simulink model "RealtimeModel"  (Simulink 7.0)
settings: Solver=FixedStepDiscrete  SolverMode=MultiTasking  StartTime=0.0  StopTime=RunningTime  FixedStep=sample  RelTol=1e-3
undefined symbols (not defined in the file): Elements, Integrator, SampleRate, Structure
libraries: simulink x2
(part 1 of 3)
settings Model: Creator=Tommy  LastModifiedBy=Tommy  BufferReuse=off
settings OptimizationCC: BlockReduction=off  OptimizeBlockIOStorage=off  BufferReuse=off  ExpressionFolding=off  LocalBlockOutputs=off
settings RTWCC: SystemTargetFile=xpctarget.tlc  TemplateMakefile=xpc_default_tmf  Description=xPC Target  ProcessScript=xpctarget_make_rtw_hook
settings xpcTargetCC: TargetFcnLib=ansi_tfl_table_tmw.mat  GenFloatMathFcnCalls=ANSI_C  CompOptLevelCompliant=off  PortableWordSizes=off
settings CustomProperty: DataType=string  Value=Real-Time

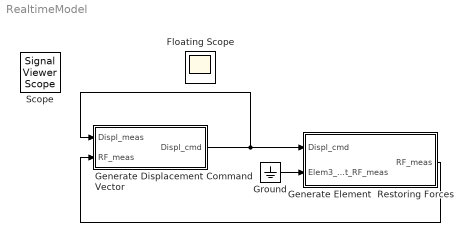
== system RealtimeModel ==
  Generate Displacement Command Vector : Subsystem
      mask Type: Generate Displacement Command Vector
      mask Description:
      | Generates the Displacement vector using the CR Algorithm.
      | 
      | Connect the measured displacement vector and measured restoring force vector to the inputs.
  Generate Element  Restoring Forces : Subsystem  TreatAsAtomicUnit=on  SystemSampleTime=SampleRate
  Ground : Ground
  Floating Scope : Scope
      settings: Floating=on
  Scope : SignalViewerScope  IOType=viewer  SampleTime=-1  RefreshTime=0.035000
  wires:
  Generate Displacement Command Vector/1(Displ_cmd) -> Generate Element  Restoring Forces/1(Displ_cmd), Generate Displacement Command Vector/1(Displ_meas)
  Generate Element  Restoring Forces/1(RF_meas) -> Generate Displacement Command Vector/2(RF_meas)
  Ground/1 -> Generate Element  Restoring Forces/2(Elem3_Act_RF_meas)

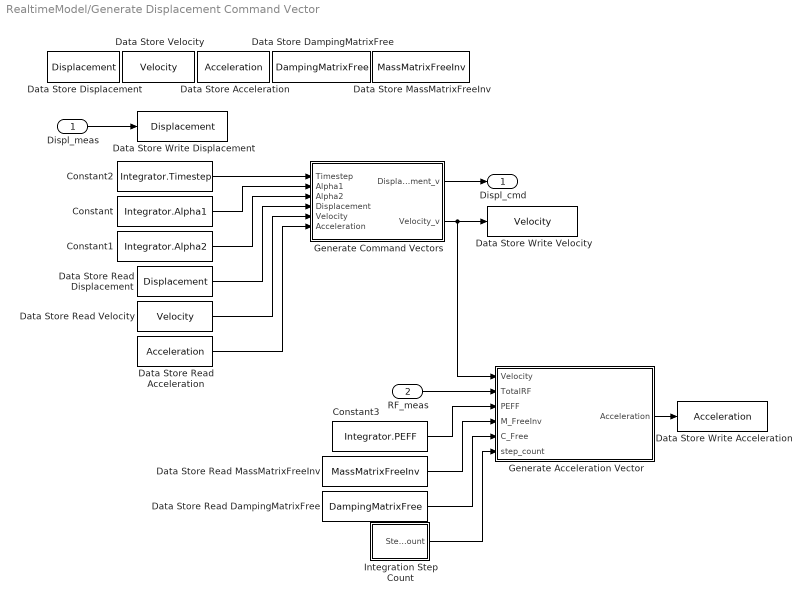
== system RealtimeModel/Generate Displacement Command Vector ==
  Displ_meas : Inport  OutDataType=sfix(16)  OutScaling=2^0
  RF_meas : Inport  Port=2  OutDataType=sfix(16)  OutScaling=2^0
  Constant : Constant  Value=Integrator.Alpha1  OutDataType=sfix(16)  OutScaling=2^0
  Constant1 : Constant  Value=Integrator.Alpha2  OutDataType=sfix(16)  OutScaling=2^0
  Constant2 : Constant  Value=Integrator.Timestep  OutDataType=sfix(16)  OutScaling=2^0
  Constant3 : Constant  Value=Integrator.PEFF  OutDataType=sfix(16)  OutScaling=2^0
  Data Store Acceleration : DataStoreMemory  DataStoreName=Acceleration  InitialValue=Integrator.Acceleration  OutDataType=sfix(16)  OutScaling=2^0
  Data Store DampingMatrixFree : DataStoreMemory  DataStoreName=DampingMatrixFree  InitialValue=Structure.DampingMatrixFree  OutDataType=sfix(16)  OutScaling=2^0
  Data Store Displacement : DataStoreMemory  DataStoreName=Displacement  InitialValue=Integrator.Displacement  OutDataType=sfix(16)  OutScaling=2^0
  Data Store MassMatrixFreeInv : DataStoreMemory  DataStoreName=MassMatrixFreeInv  InitialValue=Structure.MassMatrixFreeInv  OutDataType=sfix(16)  OutScaling=2^0
  Data Store Read Acceleration : DataStoreRead  DataStoreName=Acceleration  SampleTime=SampleRate
  Data Store Read DampingMatrixFree : DataStoreRead  DataStoreName=DampingMatrixFree  SampleTime=SampleRate
  Data Store Read Displacement : DataStoreRead  DataStoreName=Displacement  SampleTime=SampleRate
  Data Store Read MassMatrixFreeInv : DataStoreRead  DataStoreName=MassMatrixFreeInv  SampleTime=SampleRate
  Data Store Read Velocity : DataStoreRead  DataStoreName=Velocity  SampleTime=SampleRate
  Data Store Velocity : DataStoreMemory  DataStoreName=Velocity  InitialValue=Integrator.Velocity  OutDataType=sfix(16)  OutScaling=2^0
  Data Store Write Acceleration : DataStoreWrite  DataStoreName=Acceleration  SampleTime=-1
  Data Store Write Displacement : DataStoreWrite  DataStoreName=Displacement  SampleTime=-1
  Data Store Write Velocity : DataStoreWrite  DataStoreName=Velocity  SampleTime=-1
  Generate Acceleration Vector : Stateflow chart  TreatAsAtomicUnit=on  SystemSampleTime=SampleRate
  Generate Command Vectors : Stateflow chart  TreatAsAtomicUnit=on  SystemSampleTime=SampleRate
  Integration Step Count : Subsystem  TreatAsAtomicUnit=on  SystemSampleTime=SampleRate
      mask Type: Step count
      mask Description: Generates the step count
  Displ_cmd : Outport  OutDataType=sfix(16)  OutScaling=2^0
  wires:
  Generate Command Vectors/1(Displacement_v) -> Displ_cmd/1
  Constant2/1 -> Generate Command Vectors/1(Timestep)
  Constant1/1 -> Generate Command Vectors/3(Alpha2)
  Data Store Read Displacement/1 -> Generate Command Vectors/4(Displacement)
  Data Store Read Velocity/1 -> Generate Command Vectors/5(Velocity)
  Data Store Read Acceleration/1 -> Generate Command Vectors/6(Acceleration)
  Constant/1 -> Generate Command Vectors/2(Alpha1)
  Displ_meas/1 -> Data Store Write Displacement/1
  RF_meas/1 -> Generate Acceleration Vector/2(TotalRF)
  Generate Command Vectors/2(Velocity_v) -> Data Store Write Velocity/1, Generate Acceleration Vector/1(Velocity)
  Generate Acceleration Vector/1(Acceleration) -> Data Store Write Acceleration/1
  Constant3/1 -> Generate Acceleration Vector/3(PEFF)
  Data Store Read MassMatrixFreeInv/1 -> Generate Acceleration Vector/4(M_FreeInv)
  Data Store Read DampingMatrixFree/1 -> Generate Acceleration Vector/5(C_Free)
  Integration Step Count/1(Step Count) -> Generate Acceleration Vector/6(step_count)

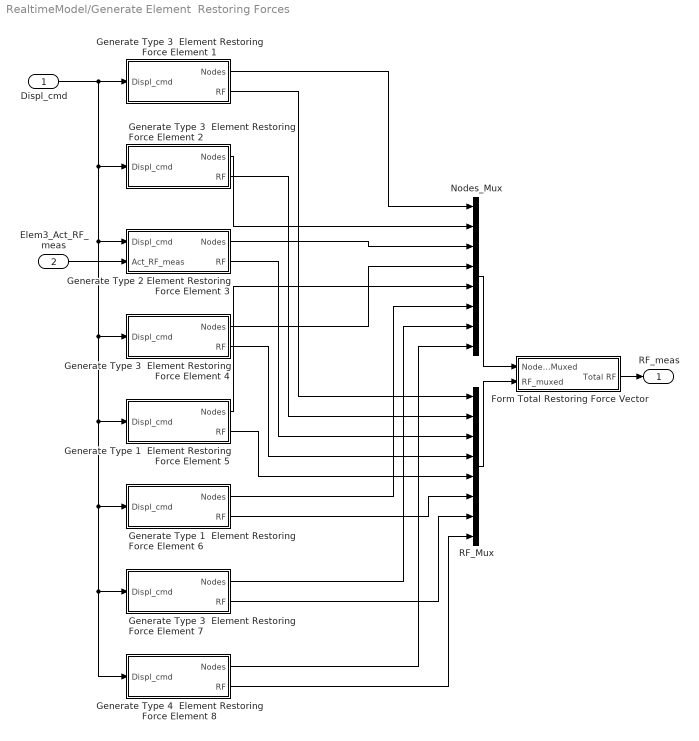
== system RealtimeModel/Generate Element  Restoring Forces ==
  Displ_cmd : Inport  OutDataType=sfix(16)  OutScaling=2^0
  Elem3_Act_RF_meas : Inport  Port=2  OutDataType=sfix(16)  OutScaling=2^0
  Form Total Restoring Force Vector : Subsystem  TreatAsAtomicUnit=on  SystemSampleTime=SampleRate
      mask Type: Form Restoring Force Vector
      mask Description:
      | Takes the restoring force vectors from each Element and combines them to form a total restoring force vector.
      | 
      | Connect the "Nodes_muxed" signal to the output of a Mux block which takes in all the Element "Nodes" outputs in order of ID.
      | 
      | Connect the "RF_muxed" signal to the output of a Mux block which takes in all the Element "RF" outputs in order of ID.
  Generate Type 1  Element Restoring Force Element 5 : Subsystem  TreatAsAtomicUnit=on  SystemSampleTime=SampleRate  mask(Generate Type 1 Element Restoring Force){id=5}
      mask prompts: id "Element ID"
      mask help:
      | Generates the Restoring Force vector for a Type 1 Element
      |
      | Enter the ID for this element corresponding with the input configuration file
  Generate Type 1  Element Restoring Force Element 6 : Subsystem  TreatAsAtomicUnit=on  SystemSampleTime=SampleRate  mask(Generate Type 1 Element Restoring Force){id=6}
      mask prompts: id "Element ID"
      mask help:
      | Generates the Restoring Force vector for a Type 1 Element
      |
      | Enter the ID for this element corresponding with the input configuration file
  Generate Type 2 Element Restoring Force Element 3 : Subsystem  TreatAsAtomicUnit=on  SystemSampleTime=SampleRate  mask(Generate Type 2 Element Restoring Force){id=3, simulation=off}
      mask prompts: id "Element ID"; simulation "Experiment Mode"
      mask help:
      | Generates the Restoring Force vector for a Type 2 Element
      |
      | Enter the ID for this element corresponding with the input configuration file
      |
      | Check the "Experiment Mode" box to activate the Act_RF_meas input.
      | Connect the Actuator Restoring Force feedback to the input.
  Generate Type 3  Element Restoring Force Element 1 : Subsystem  TreatAsAtomicUnit=on  SystemSampleTime=SampleRate  mask(Generate Type 3 Element Restoring Force){id=1}
      mask prompts: id "Element ID"
      mask help:
      | Generates the Restoring Force vector for a Type 3 Element
      |
      | Enter the ID for this element corresponding with the input configuration file
  Generate Type 3  Element Restoring Force Element 2 : Subsystem  TreatAsAtomicUnit=on  SystemSampleTime=SampleRate  mask(Generate Type 3 Element Restoring Force){id=2}
      mask prompts: id "Element ID"
      mask help:
      | Generates the Restoring Force vector for a Type 3 Element
      |
      | Enter the ID for this element corresponding with the input configuration file
  Generate Type 3  Element Restoring Force Element 4 : Subsystem  TreatAsAtomicUnit=on  SystemSampleTime=SampleRate  mask(Generate Type 3 Element Restoring Force){id=4}
      mask prompts: id "Element ID"
      mask help:
      | Generates the Restoring Force vector for a Type 3 Element
      |
      | Enter the ID for this element corresponding with the input configuration file
  Generate Type 3  Element Restoring Force Element 7 : Subsystem  TreatAsAtomicUnit=on  SystemSampleTime=SampleRate  mask(Generate Type 3 Element Restoring Force){id=7}
      mask prompts: id "Element ID"
      mask help:
      | Generates the Restoring Force vector for a Type 3 Element
      |
      | Enter the ID for this element corresponding with the input configuration file
  Generate Type 4  Element Restoring Force Element 8 : Subsystem  TreatAsAtomicUnit=on  SystemSampleTime=SampleRate  mask(Generate Type 4 Element Restoring Force){id=8}
      mask prompts: id "Element ID"
      mask help:
      | Generates the Restoring Force vector for a Type 4 Element
      |
      | Enter the ID for this element corresponding with the input configuration file
  Nodes_Mux : Mux  Inputs=8
  RF_Mux : Mux  Inputs=8
  RF_meas : Outport  OutDataType=sfix(16)  OutScaling=2^0
  wires:
  Displ_cmd/1 -> Generate Type 3  Element Restoring Force Element 1/1(Displ_cmd), Generate Type 3  Element Restoring Force Element 2/1(Displ_cmd), Generate Type 2 Element Restoring Force Element 3/1(Displ_cmd), Generate Type 3  Element Restoring Force Element 4/1(Displ_cmd), Generate Type 1  Element Restoring Force Element 5/1(Displ_cmd), Generate Type 1  Element Restoring Force Element 6/1(Displ_cmd), Generate Type 3  Element Restoring Force Element 7/1(Displ_cmd), Generate Type 4  Element Restoring Force Element 8/1(Displ_cmd)
  Generate Type 3  Element Restoring Force Element 1/1(Nodes) -> Nodes_Mux/1
  Generate Type 3  Element Restoring Force Element 2/1(Nodes) -> Nodes_Mux/2
  Generate Type 2 Element Restoring Force Element 3/1(Nodes) -> Nodes_Mux/3
  Generate Type 3  Element Restoring Force Element 4/1(Nodes) -> Nodes_Mux/4
  Generate Type 1  Element Restoring Force Element 5/1(Nodes) -> Nodes_Mux/5
  Generate Type 1  Element Restoring Force Element 6/1(Nodes) -> Nodes_Mux/6
  Generate Type 3  Element Restoring Force Element 7/1(Nodes) -> Nodes_Mux/7
  Generate Type 4  Element Restoring Force Element 8/1(Nodes) -> Nodes_Mux/8
  Generate Type 3  Element Restoring Force Element 1/2(RF) -> RF_Mux/1
  Generate Type 3  Element Restoring Force Element 2/2(RF) -> RF_Mux/2
  Generate Type 2 Element Restoring Force Element 3/2(RF) -> RF_Mux/3
  Generate Type 3  Element Restoring Force Element 4/2(RF) -> RF_Mux/4
  Generate Type 1  Element Restoring Force Element 5/2(RF) -> RF_Mux/5
  Generate Type 1  Element Restoring Force Element 6/2(RF) -> RF_Mux/6
  Generate Type 3  Element Restoring Force Element 7/2(RF) -> RF_Mux/7
  Generate Type 4  Element Restoring Force Element 8/2(RF) -> RF_Mux/8
  Form Total Restoring Force Vector/1(Total RF) -> RF_meas/1
  Nodes_Mux/1 -> Form Total Restoring Force Vector/1(Nodes_Muxed)
  RF_Mux/1 -> Form Total Restoring Force Vector/2(RF_muxed)
  Elem3_Act_RF_meas/1 -> Generate Type 2 Element Restoring Force Element 3/2(Act_RF_meas)

== system RealtimeModel/Generate Displacement Command Vector/Integration Step Count ==
  Increment Stored Integer : simulink/Additional Math & Discrete/Additional Math: Increment - Decrement/Increment Stored Integer  SystemSampleTime=-1
  step count : simulink/Sources/Counter Free-Running  SystemSampleTime=-1  NumBits=32  tsamp=-1
  Step Count : Outport  OutDataType=sfix(16)  OutScaling=2^0
  wires:
  step count/1 -> Increment Stored Integer/1
  Increment Stored Integer/1 -> Step Count/1

== system RealtimeModel/Generate Element  Restoring Forces/Form Total Restoring Force Vector ==
  Nodes_Muxed : Inport  OutDataType=sfix(16)  OutScaling=2^0
  RF_muxed : Inport  Port=2  OutDataType=sfix(16)  OutScaling=2^0
  Form Restoring Force Vector : Stateflow chart  TreatAsAtomicUnit=on  SystemSampleTime=SampleRate
  Total RF : Outport  OutDataType=sfix(16)  OutScaling=2^0
  wires:
  RF_muxed/1 -> Form Restoring Force Vector/2(RF_muxed)
  Form Restoring Force Vector/1(TotalRF) -> Total RF/1
  Nodes_Muxed/1 -> Form Restoring Force Vector/1(Nodes_muxed)

== system RealtimeModel/Generate Element  Restoring Forces/Generate Type 1  Element Restoring Force Element 5 ==
  Displ_cmd : Inport  OutDataType=sfix(16)  OutScaling=2^0
  Constant : Constant  Value=Structure.NumFreeDOF  OutDataType=sfix(16)  OutScaling=2^0
  "Type 1 Element " : Subsystem  mask(Element Type 1){id=id}
      mask prompts: id "Element ID:"
      mask help: Enter the ID for this element corresponding with the input configuration file
  Type 1 Element RF : Stateflow chart  TreatAsAtomicUnit=on  SystemSampleTime=SampleRate
  Nodes : Outport  OutDataType=sfix(16)  OutScaling=2^0
  RF : Outport  Port=2  OutDataType=sfix(16)  OutScaling=2^0
  wires:
  "Type 1 Element "/1(Element) -> Type 1 Element RF/1(Element)
  Displ_cmd/1 -> Type 1 Element RF/3(Displacement)
  Type 1 Element RF/2(RF) -> RF/1
  Type 1 Element RF/1(Nodes) -> Nodes/1
  Constant/1 -> Type 1 Element RF/2(NumFreeDOF)

== system RealtimeModel/Generate Element  Restoring Forces/Generate Type 1  Element Restoring Force Element 6 ==
  Displ_cmd : Inport  OutDataType=sfix(16)  OutScaling=2^0
  Constant : Constant  Value=Structure.NumFreeDOF  OutDataType=sfix(16)  OutScaling=2^0
  "Type 1 Element " : Subsystem  mask(Element Type 1){id=id}
      mask prompts: id "Element ID:"
      mask help: Enter the ID for this element corresponding with the input configuration file
  Type 1 Element RF : Stateflow chart  TreatAsAtomicUnit=on  SystemSampleTime=SampleRate
  Nodes : Outport  OutDataType=sfix(16)  OutScaling=2^0
  RF : Outport  Port=2  OutDataType=sfix(16)  OutScaling=2^0
  wires:
  Constant/1 -> Type 1 Element RF/2(NumFreeDOF)
  Type 1 Element RF/1(Nodes) -> Nodes/1
  Type 1 Element RF/2(RF) -> RF/1
  Displ_cmd/1 -> Type 1 Element RF/3(Displacement)
  "Type 1 Element "/1(Element) -> Type 1 Element RF/1(Element)

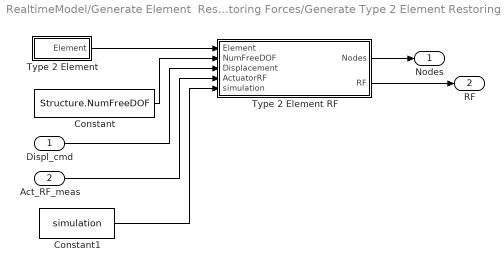
== system RealtimeModel/Generate Element  Restoring Forces/Generate Type 2 Element Restoring Force Element 3 ==
  Displ_cmd : Inport  OutDataType=sfix(16)  OutScaling=2^0
  Act_RF_meas : Inport  Port=2  OutDataType=sfix(16)  OutScaling=2^0
  Constant : Constant  Value=Structure.NumFreeDOF  OutDataType=sfix(16)  OutScaling=2^0
  Constant1 : Constant  Value=simulation  OutDataType=sfix(16)  OutScaling=2^0
  Type 2 Element : Subsystem  mask(Element Type 2){id=id}
      mask prompts: id "Element ID:"
      mask help: Enter the ID for this element corresponding with the input configuration file
  Type 2 Element RF : Stateflow chart  TreatAsAtomicUnit=on  SystemSampleTime=SampleRate
  Nodes : Outport  OutDataType=sfix(16)  OutScaling=2^0
  RF : Outport  Port=2  OutDataType=sfix(16)  OutScaling=2^0
  wires:
  Type 2 Element/1(Element) -> Type 2 Element RF/1(Element)
  Act_RF_meas/1 -> Type 2 Element RF/4(ActuatorRF)
  Type 2 Element RF/1(Nodes) -> Nodes/1
  Type 2 Element RF/2(RF) -> RF/1
  Displ_cmd/1 -> Type 2 Element RF/3(Displacement)
  Constant/1 -> Type 2 Element RF/2(NumFreeDOF)
  Constant1/1 -> Type 2 Element RF/5(simulation)

== system RealtimeModel/Generate Element  Restoring Forces/Generate Type 3  Element Restoring Force Element 1 ==
  Displ_cmd : Inport  OutDataType=sfix(16)  OutScaling=2^0
  Constant : Constant  Value=Structure.NumFreeDOF  OutDataType=sfix(16)  OutScaling=2^0
  "Type 3 Element " : Subsystem  mask(Element Type 3){id=id}
      mask prompts: id "Element ID:"
      mask help: Enter the ID for this element corresponding with the input configuration file
  Type 3 Element RF : Stateflow chart  TreatAsAtomicUnit=on  SystemSampleTime=SampleRate
  Nodes : Outport  OutDataType=sfix(16)  OutScaling=2^0
  RF : Outport  Port=2  OutDataType=sfix(16)  OutScaling=2^0
  wires:
  "Type 3 Element "/5(bmy) -> Type 3 Element RF/5(bmy_init)
  "Type 3 Element "/4(pmx) -> Type 3 Element RF/4(pmx)
  "Type 3 Element "/3(a2) -> Type 3 Element RF/3(a2)
  "Type 3 Element "/2(a1) -> Type 3 Element RF/2(a1)
  Type 3 Element RF/1(Nodes) -> Nodes/1
  Type 3 Element RF/2(RF) -> RF/1
  "Type 3 Element "/1(Element) -> Type 3 Element RF/1(Element)
  Displ_cmd/1 -> Type 3 Element RF/7(Displacement)
  Constant/1 -> Type 3 Element RF/6(NumFreeDOF)

== system RealtimeModel/Generate Element  Restoring Forces/Generate Type 3  Element Restoring Force Element 2 ==
  Displ_cmd : Inport  OutDataType=sfix(16)  OutScaling=2^0
  Constant : Constant  Value=Structure.NumFreeDOF  OutDataType=sfix(16)  OutScaling=2^0
  "Type 3 Element " : Subsystem  mask(Element Type 3){id=id}
      mask prompts: id "Element ID:"
      mask help: Enter the ID for this element corresponding with the input configuration file
  Type 3 Element RF : Stateflow chart  TreatAsAtomicUnit=on  SystemSampleTime=SampleRate
  Nodes : Outport  OutDataType=sfix(16)  OutScaling=2^0
  RF : Outport  Port=2  OutDataType=sfix(16)  OutScaling=2^0
  wires:
  Constant/1 -> Type 3 Element RF/6(NumFreeDOF)
  Displ_cmd/1 -> Type 3 Element RF/7(Displacement)
  "Type 3 Element "/1(Element) -> Type 3 Element RF/1(Element)
  Type 3 Element RF/2(RF) -> RF/1
  Type 3 Element RF/1(Nodes) -> Nodes/1
  "Type 3 Element "/2(a1) -> Type 3 Element RF/2(a1)
  "Type 3 Element "/3(a2) -> Type 3 Element RF/3(a2)
  "Type 3 Element "/4(pmx) -> Type 3 Element RF/4(pmx)
  "Type 3 Element "/5(bmy) -> Type 3 Element RF/5(bmy_init)

== system RealtimeModel/Generate Element  Restoring Forces/Generate Type 3  Element Restoring Force Element 4 ==
  Displ_cmd : Inport  OutDataType=sfix(16)  OutScaling=2^0
  Constant : Constant  Value=Structure.NumFreeDOF  OutDataType=sfix(16)  OutScaling=2^0
  "Type 3 Element " : Subsystem  mask(Element Type 3){id=id}
      mask prompts: id "Element ID:"
      mask help: Enter the ID for this element corresponding with the input configuration file
  Type 3 Element RF : Stateflow chart  TreatAsAtomicUnit=on  SystemSampleTime=SampleRate
  Nodes : Outport  OutDataType=sfix(16)  OutScaling=2^0
  RF : Outport  Port=2  OutDataType=sfix(16)  OutScaling=2^0
  wires:
  "Type 3 Element "/5(bmy) -> Type 3 Element RF/5(bmy_init)
  "Type 3 Element "/4(pmx) -> Type 3 Element RF/4(pmx)
  "Type 3 Element "/3(a2) -> Type 3 Element RF/3(a2)
  "Type 3 Element "/2(a1) -> Type 3 Element RF/2(a1)
  Type 3 Element RF/1(Nodes) -> Nodes/1
  Type 3 Element RF/2(RF) -> RF/1
  "Type 3 Element "/1(Element) -> Type 3 Element RF/1(Element)
  Displ_cmd/1 -> Type 3 Element RF/7(Displacement)
  Constant/1 -> Type 3 Element RF/6(NumFreeDOF)

== system RealtimeModel/Generate Element  Restoring Forces/Generate Type 3  Element Restoring Force Element 7 ==
  Displ_cmd : Inport  OutDataType=sfix(16)  OutScaling=2^0
  Constant : Constant  Value=Structure.NumFreeDOF  OutDataType=sfix(16)  OutScaling=2^0
  "Type 3 Element " : Subsystem  mask(Element Type 3){id=id}
      mask prompts: id "Element ID:"
      mask help: Enter the ID for this element corresponding with the input configuration file
  Type 3 Element RF : Stateflow chart  TreatAsAtomicUnit=on  SystemSampleTime=SampleRate
  Nodes : Outport  OutDataType=sfix(16)  OutScaling=2^0
  RF : Outport  Port=2  OutDataType=sfix(16)  OutScaling=2^0
  wires:
  Constant/1 -> Type 3 Element RF/6(NumFreeDOF)
  Displ_cmd/1 -> Type 3 Element RF/7(Displacement)
  "Type 3 Element "/1(Element) -> Type 3 Element RF/1(Element)
  Type 3 Element RF/2(RF) -> RF/1
  Type 3 Element RF/1(Nodes) -> Nodes/1
  "Type 3 Element "/2(a1) -> Type 3 Element RF/2(a1)
  "Type 3 Element "/3(a2) -> Type 3 Element RF/3(a2)
  "Type 3 Element "/4(pmx) -> Type 3 Element RF/4(pmx)
  "Type 3 Element "/5(bmy) -> Type 3 Element RF/5(bmy_init)

== system RealtimeModel/Generate Element  Restoring Forces/Generate Type 4  Element Restoring Force Element 8 ==
  Displ_cmd : Inport  OutDataType=sfix(16)  OutScaling=2^0
  Constant : Constant  Value=Structure.NumFreeDOF  OutDataType=sfix(16)  OutScaling=2^0
  "Type 4 Element " : Subsystem  mask(Element Type 4){id=id}
      mask prompts: id "Element ID:"
      mask help: Enter the ID for this element corresponding with the input configuration file
  Type 4 Element RF : Stateflow chart  TreatAsAtomicUnit=on  SystemSampleTime=SampleRate
  Nodes : Outport  OutDataType=sfix(16)  OutScaling=2^0
  RF : Outport  Port=2  OutDataType=sfix(16)  OutScaling=2^0
  wires:
  "Type 4 Element "/1(Element) -> Type 4 Element RF/1(Element)
  Type 4 Element RF/1(Nodes) -> Nodes/1
  Type 4 Element RF/2(RF) -> RF/1
  Constant/1 -> Type 4 Element RF/2(NumFreeDOF)
  Displ_cmd/1 -> Type 4 Element RF/3(Displacement)

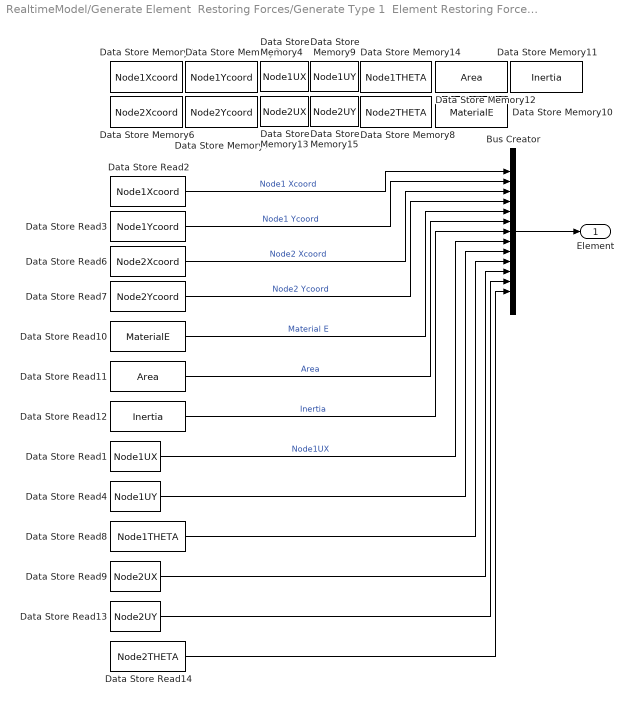
== system RealtimeModel/Generate Element  Restoring Forces/Generate Type 1  Element Restoring Force Element 5/Type 1 Element  ==
  Bus Creator : BusCreator  Inputs=13
  Data Store Memory10 : DataStoreMemory  DataStoreName=MaterialE  InitialValue=Elements{id}.Material(1).E  OutDataType=sfix(16)  OutScaling=2^0
  Data Store Memory11 : DataStoreMemory  DataStoreName=Inertia  InitialValue=Elements{id}.Inertia  OutDataType=sfix(16)  OutScaling=2^0
  Data Store Memory12 : DataStoreMemory  DataStoreName=Area  InitialValue=Elements{id}.Area  OutDataType=sfix(16)  OutScaling=2^0
  Data Store Memory13 : DataStoreMemory  DataStoreName=Node2UX  InitialValue=Elements{id}.Nodes(2).UX  OutDataType=sfix(16)  OutScaling=2^0
  Data Store Memory14 : DataStoreMemory  DataStoreName=Node1THETA  InitialValue=Elements{id}.Nodes(1).THETA  OutDataType=sfix(16)  OutScaling=2^0
  Data Store Memory15 : DataStoreMemory  DataStoreName=Node2UY  InitialValue=Elements{id}.Nodes(2).UY  OutDataType=sfix(16)  OutScaling=2^0
  Data Store Memory2 : DataStoreMemory  DataStoreName=Node1Xcoord  InitialValue=Elements{id}.Nodes(1).Xcoord  OutDataType=sfix(16)  OutScaling=2^0
  Data Store Memory3 : DataStoreMemory  DataStoreName=Node1Ycoord  InitialValue=Elements{id}.Nodes(1).Ycoord  OutDataType=sfix(16)  OutScaling=2^0
  Data Store Memory4 : DataStoreMemory  DataStoreName=Node1UX  InitialValue=Elements{id}.Nodes(1).UX  OutDataType=sfix(16)  OutScaling=2^0
  Data Store Memory6 : DataStoreMemory  DataStoreName=Node2Xcoord  InitialValue=Elements{id}.Nodes(2).Xcoord  OutDataType=sfix(16)  OutScaling=2^0
  Data Store Memory7 : DataStoreMemory  DataStoreName=Node2Ycoord  InitialValue=Elements{id}.Nodes(2).Ycoord  OutDataType=sfix(16)  OutScaling=2^0
  Data Store Memory8 : DataStoreMemory  DataStoreName=Node2THETA  InitialValue=Elements{id}.Nodes(2).THETA  OutDataType=sfix(16)  OutScaling=2^0
  Data Store Memory9 : DataStoreMemory  DataStoreName=Node1UY  InitialValue=Elements{id}.Nodes(1).UY  OutDataType=sfix(16)  OutScaling=2^0
  Data Store Read1 : DataStoreRead  DataStoreName=Node1UX  SampleTime=-1
  Data Store Read10 : DataStoreRead  DataStoreName=MaterialE  SampleTime=-1
  Data Store Read11 : DataStoreRead  DataStoreName=Area  SampleTime=-1
  Data Store Read12 : DataStoreRead  DataStoreName=Inertia  SampleTime=-1
  Data Store Read13 : DataStoreRead  DataStoreName=Node2UY  SampleTime=-1
  Data Store Read14 : DataStoreRead  DataStoreName=Node2THETA  SampleTime=-1
  Data Store Read2 : DataStoreRead  DataStoreName=Node1Xcoord  SampleTime=-1
  Data Store Read3 : DataStoreRead  DataStoreName=Node1Ycoord  SampleTime=-1
  Data Store Read4 : DataStoreRead  DataStoreName=Node1UY  SampleTime=-1
  Data Store Read6 : DataStoreRead  DataStoreName=Node2Xcoord  SampleTime=-1
  Data Store Read7 : DataStoreRead  DataStoreName=Node2Ycoord  SampleTime=-1
  Data Store Read8 : DataStoreRead  DataStoreName=Node1THETA  SampleTime=-1
  Data Store Read9 : DataStoreRead  DataStoreName=Node2UX  SampleTime=-1
  Element : Outport  OutDataType=sfix(16)  OutScaling=2^0
  wires:
  Data Store Read14/1 -> Bus Creator/13
  Data Store Read13/1 -> Bus Creator/12
  Data Store Read9/1 -> Bus Creator/11
  Data Store Read8/1 -> Bus Creator/10
  Data Store Read4/1 -> Bus Creator/9
  Data Store Read1/1 -> Bus Creator/8  "Node1UX"
  Data Store Read2/1 -> Bus Creator/1  "Node1 Xcoord"
  Data Store Read3/1 -> Bus Creator/2  "Node1 Ycoord"
  Data Store Read6/1 -> Bus Creator/3  "Node2 Xcoord"
  Data Store Read7/1 -> Bus Creator/4  "Node2 Ycoord"
  Data Store Read10/1 -> Bus Creator/5  "Material E"
  Data Store Read11/1 -> Bus Creator/6  "Area"
  Data Store Read12/1 -> Bus Creator/7  "Inertia"
  Bus Creator/1 -> Element/1

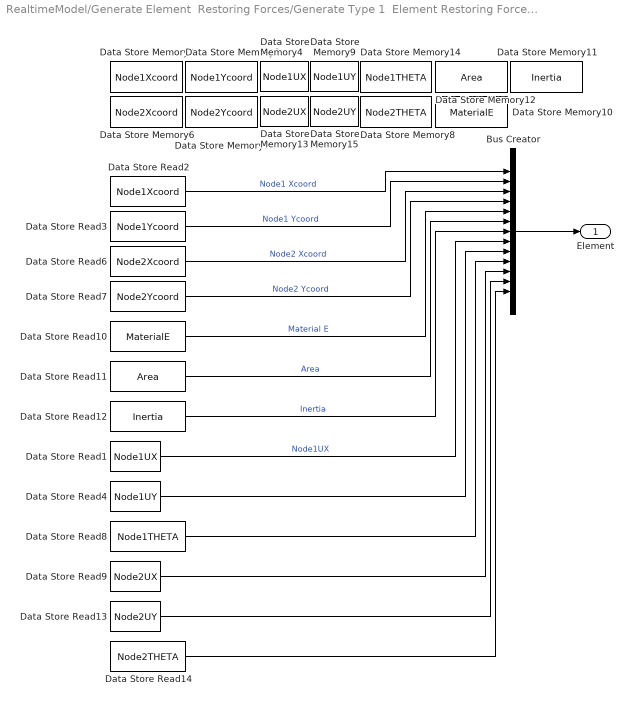
== system RealtimeModel/Generate Element  Restoring Forces/Generate Type 1  Element Restoring Force Element 6/Type 1 Element  ==
  Bus Creator : BusCreator  Inputs=13
  Data Store Memory10 : DataStoreMemory  DataStoreName=MaterialE  InitialValue=Elements{id}.Material(1).E  OutDataType=sfix(16)  OutScaling=2^0
  Data Store Memory11 : DataStoreMemory  DataStoreName=Inertia  InitialValue=Elements{id}.Inertia  OutDataType=sfix(16)  OutScaling=2^0
  Data Store Memory12 : DataStoreMemory  DataStoreName=Area  InitialValue=Elements{id}.Area  OutDataType=sfix(16)  OutScaling=2^0
  Data Store Memory13 : DataStoreMemory  DataStoreName=Node2UX  InitialValue=Elements{id}.Nodes(2).UX  OutDataType=sfix(16)  OutScaling=2^0
  Data Store Memory14 : DataStoreMemory  DataStoreName=Node1THETA  InitialValue=Elements{id}.Nodes(1).THETA  OutDataType=sfix(16)  OutScaling=2^0
  Data Store Memory15 : DataStoreMemory  DataStoreName=Node2UY  InitialValue=Elements{id}.Nodes(2).UY  OutDataType=sfix(16)  OutScaling=2^0
  Data Store Memory2 : DataStoreMemory  DataStoreName=Node1Xcoord  InitialValue=Elements{id}.Nodes(1).Xcoord  OutDataType=sfix(16)  OutScaling=2^0
  Data Store Memory3 : DataStoreMemory  DataStoreName=Node1Ycoord  InitialValue=Elements{id}.Nodes(1).Ycoord  OutDataType=sfix(16)  OutScaling=2^0
  Data Store Memory4 : DataStoreMemory  DataStoreName=Node1UX  InitialValue=Elements{id}.Nodes(1).UX  OutDataType=sfix(16)  OutScaling=2^0
  Data Store Memory6 : DataStoreMemory  DataStoreName=Node2Xcoord  InitialValue=Elements{id}.Nodes(2).Xcoord  OutDataType=sfix(16)  OutScaling=2^0
  Data Store Memory7 : DataStoreMemory  DataStoreName=Node2Ycoord  InitialValue=Elements{id}.Nodes(2).Ycoord  OutDataType=sfix(16)  OutScaling=2^0
  Data Store Memory8 : DataStoreMemory  DataStoreName=Node2THETA  InitialValue=Elements{id}.Nodes(2).THETA  OutDataType=sfix(16)  OutScaling=2^0
  Data Store Memory9 : DataStoreMemory  DataStoreName=Node1UY  InitialValue=Elements{id}.Nodes(1).UY  OutDataType=sfix(16)  OutScaling=2^0
  Data Store Read1 : DataStoreRead  DataStoreName=Node1UX  SampleTime=-1
  Data Store Read10 : DataStoreRead  DataStoreName=MaterialE  SampleTime=-1
  Data Store Read11 : DataStoreRead  DataStoreName=Area  SampleTime=-1
  Data Store Read12 : DataStoreRead  DataStoreName=Inertia  SampleTime=-1
  Data Store Read13 : DataStoreRead  DataStoreName=Node2UY  SampleTime=-1
  Data Store Read14 : DataStoreRead  DataStoreName=Node2THETA  SampleTime=-1
  Data Store Read2 : DataStoreRead  DataStoreName=Node1Xcoord  SampleTime=-1
  Data Store Read3 : DataStoreRead  DataStoreName=Node1Ycoord  SampleTime=-1
  Data Store Read4 : DataStoreRead  DataStoreName=Node1UY  SampleTime=-1
  Data Store Read6 : DataStoreRead  DataStoreName=Node2Xcoord  SampleTime=-1
  Data Store Read7 : DataStoreRead  DataStoreName=Node2Ycoord  SampleTime=-1
  Data Store Read8 : DataStoreRead  DataStoreName=Node1THETA  SampleTime=-1
  Data Store Read9 : DataStoreRead  DataStoreName=Node2UX  SampleTime=-1
  Element : Outport  OutDataType=sfix(16)  OutScaling=2^0
  wires:
  Bus Creator/1 -> Element/1
  Data Store Read12/1 -> Bus Creator/7  "Inertia"
  Data Store Read11/1 -> Bus Creator/6  "Area"
  Data Store Read10/1 -> Bus Creator/5  "Material E"
  Data Store Read7/1 -> Bus Creator/4  "Node2 Ycoord"
  Data Store Read6/1 -> Bus Creator/3  "Node2 Xcoord"
  Data Store Read3/1 -> Bus Creator/2  "Node1 Ycoord"
  Data Store Read2/1 -> Bus Creator/1  "Node1 Xcoord"
  Data Store Read1/1 -> Bus Creator/8  "Node1UX"
  Data Store Read4/1 -> Bus Creator/9
  Data Store Read8/1 -> Bus Creator/10
  Data Store Read9/1 -> Bus Creator/11
  Data Store Read13/1 -> Bus Creator/12
  Data Store Read14/1 -> Bus Creator/13

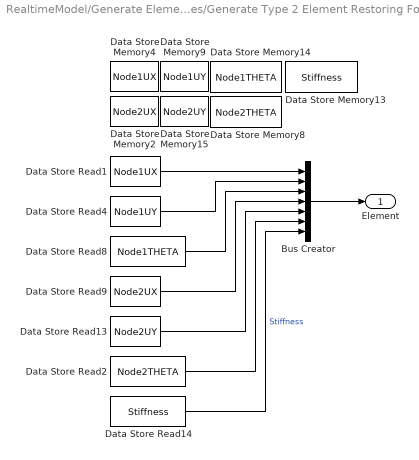
== system RealtimeModel/Generate Element  Restoring Forces/Generate Type 2 Element Restoring Force Element 3/Type 2 Element ==
  Bus Creator : BusCreator  Inputs=7
  Data Store Memory13 : DataStoreMemory  DataStoreName=Stiffness  InitialValue=Elements{id}.Stiffness  OutDataType=sfix(16)  OutScaling=2^0
  Data Store Memory14 : DataStoreMemory  DataStoreName=Node1THETA  InitialValue=Elements{id}.Nodes(1).THETA  OutDataType=sfix(16)  OutScaling=2^0
  Data Store Memory15 : DataStoreMemory  DataStoreName=Node2UY  InitialValue=Elements{id}.Nodes(2).UY  OutDataType=sfix(16)  OutScaling=2^0
  Data Store Memory2 : DataStoreMemory  DataStoreName=Node2UX  InitialValue=Elements{id}.Nodes(2).UX  OutDataType=sfix(16)  OutScaling=2^0
  Data Store Memory4 : DataStoreMemory  DataStoreName=Node1UX  InitialValue=Elements{id}.Nodes(1).UX  OutDataType=sfix(16)  OutScaling=2^0
  Data Store Memory8 : DataStoreMemory  DataStoreName=Node2THETA  InitialValue=Elements{id}.Nodes(2).THETA  OutDataType=sfix(16)  OutScaling=2^0
  Data Store Memory9 : DataStoreMemory  DataStoreName=Node1UY  InitialValue=Elements{id}.Nodes(1).UY  OutDataType=sfix(16)  OutScaling=2^0
  Data Store Read1 : DataStoreRead  DataStoreName=Node1UX  SampleTime=-1
  Data Store Read13 : DataStoreRead  DataStoreName=Node2UY  SampleTime=-1
  Data Store Read14 : DataStoreRead  DataStoreName=Stiffness  SampleTime=-1
  Data Store Read2 : DataStoreRead  DataStoreName=Node2THETA  SampleTime=-1
  Data Store Read4 : DataStoreRead  DataStoreName=Node1UY  SampleTime=-1
  Data Store Read8 : DataStoreRead  DataStoreName=Node1THETA  SampleTime=-1
  Data Store Read9 : DataStoreRead  DataStoreName=Node2UX  SampleTime=-1
  Element : Outport  OutDataType=sfix(16)  OutScaling=2^0
  wires:
  Data Store Read1/1 -> Bus Creator/1
  Data Store Read4/1 -> Bus Creator/2
  Data Store Read8/1 -> Bus Creator/3
  Data Store Read9/1 -> Bus Creator/4
  Data Store Read13/1 -> Bus Creator/5
  Data Store Read2/1 -> Bus Creator/6
  Data Store Read14/1 -> Bus Creator/7  "Stiffness"
  Bus Creator/1 -> Element/1

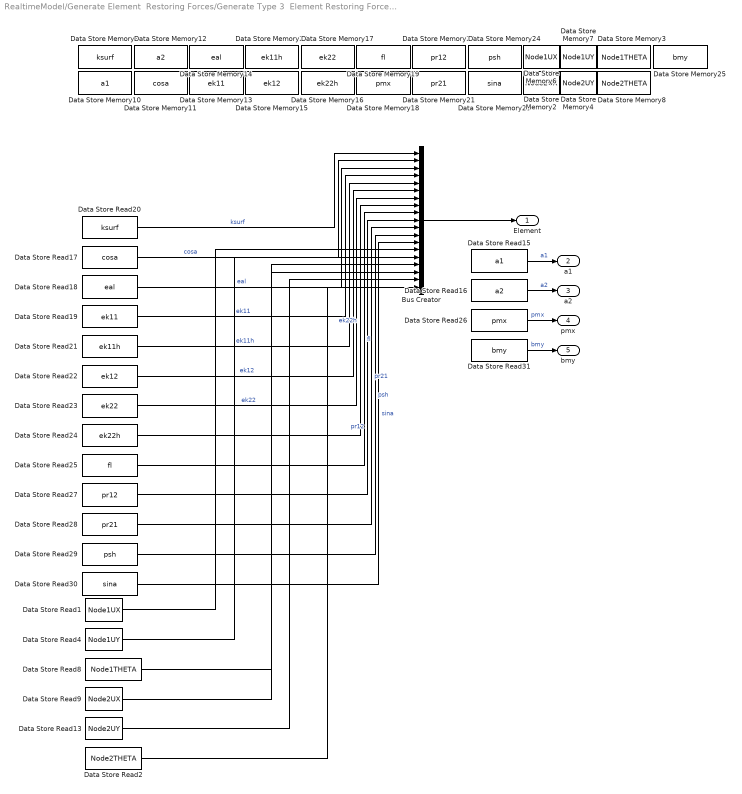
== system RealtimeModel/Generate Element  Restoring Forces/Generate Type 3  Element Restoring Force Element 1/Type 3 Element  ==
  Bus Creator : BusCreator  Inputs=19
  Data Store Memory10 : DataStoreMemory  DataStoreName=a1  InitialValue=Elements{id}.a1  OutDataType=sfix(16)  OutScaling=2^0
  Data Store Memory11 : DataStoreMemory  DataStoreName=cosa  InitialValue=Elements{id}.cosa  OutDataType=sfix(16)  OutScaling=2^0
  Data Store Memory12 : DataStoreMemory  DataStoreName=a2  InitialValue=Elements{id}.a2  OutDataType=sfix(16)  OutScaling=2^0
  Data Store Memory13 : DataStoreMemory  DataStoreName=ek11  InitialValue=Elements{id}.ek11  OutDataType=sfix(16)  OutScaling=2^0
  Data Store Memory14 : DataStoreMemory  DataStoreName=eal  InitialValue=Elements{id}.eal  OutDataType=sfix(16)  OutScaling=2^0
  Data Store Memory15 : DataStoreMemory  DataStoreName=ek12  InitialValue=Elements{id}.ek12  OutDataType=sfix(16)  OutScaling=2^0
  Data Store Memory16 : DataStoreMemory  DataStoreName=ek22h  InitialValue=Elements{id}.ek22h  OutDataType=sfix(16)  OutScaling=2^0
  Data Store Memory17 : DataStoreMemory  DataStoreName=ek22  InitialValue=Elements{id}.ek22  OutDataType=sfix(16)  OutScaling=2^0
  Data Store Memory18 : DataStoreMemory  DataStoreName=pmx  InitialValue=Elements{id}.pmx  OutDataType=sfix(16)  OutScaling=2^0
  Data Store Memory19 : DataStoreMemory  DataStoreName=fl  InitialValue=Elements{id}.fl  OutDataType=sfix(16)  OutScaling=2^0
  Data Store Memory2 : DataStoreMemory  DataStoreName=Node2UX  InitialValue=Elements{id}.Nodes(2).UX  OutDataType=sfix(16)  OutScaling=2^0
  Data Store Memory20 : DataStoreMemory  DataStoreName=ek11h  InitialValue=Elements{id}.ek11h  OutDataType=sfix(16)  OutScaling=2^0
  Data Store Memory21 : DataStoreMemory  DataStoreName=pr21  InitialValue=Elements{id}.pr21  OutDataType=sfix(16)  OutScaling=2^0
  Data Store Memory22 : DataStoreMemory  DataStoreName=pr12  InitialValue=Elements{id}.pr12  OutDataType=sfix(16)  OutScaling=2^0
  Data Store Memory23 : DataStoreMemory  DataStoreName=sina  InitialValue=Elements{id}.sina  OutDataType=sfix(16)  OutScaling=2^0
  Data Store Memory24 : DataStoreMemory  DataStoreName=psh  InitialValue=Elements{id}.psh  OutDataType=sfix(16)  OutScaling=2^0
  Data Store Memory25 : DataStoreMemory  DataStoreName=bmy  InitialValue=Elements{id}.bmy  OutDataType=sfix(16)  OutScaling=2^0
  Data Store Memory3 : DataStoreMemory  DataStoreName=Node1THETA  InitialValue=Elements{id}.Nodes(1).THETA  OutDataType=sfix(16)  OutScaling=2^0
  Data Store Memory4 : DataStoreMemory  DataStoreName=Node2UY  InitialValue=Elements{id}.Nodes(2).UY  OutDataType=sfix(16)  OutScaling=2^0
  Data Store Memory6 : DataStoreMemory  DataStoreName=Node1UX  InitialValue=Elements{id}.Nodes(1).UX  OutDataType=sfix(16)  OutScaling=2^0
  Data Store Memory7 : DataStoreMemory  DataStoreName=Node1UY  InitialValue=Elements{id}.Nodes(1).UY  OutDataType=sfix(16)  OutScaling=2^0
  Data Store Memory8 : DataStoreMemory  DataStoreName=Node2THETA  InitialValue=Elements{id}.Nodes(2).THETA  OutDataType=sfix(16)  OutScaling=2^0
  Data Store Memory9 : DataStoreMemory  DataStoreName=ksurf  InitialValue=Elements{id}.ksurf  OutDataType=sfix(16)  OutScaling=2^0
  Data Store Read1 : DataStoreRead  DataStoreName=Node1UX  SampleTime=-1
  Data Store Read13 : DataStoreRead  DataStoreName=Node2UY  SampleTime=-1
  Data Store Read15 : DataStoreRead  DataStoreName=a1  SampleTime=-1
  Data Store Read16 : DataStoreRead  DataStoreName=a2  SampleTime=-1
  Data Store Read17 : DataStoreRead  DataStoreName=cosa  SampleTime=-1
  Data Store Read18 : DataStoreRead  DataStoreName=eal  SampleTime=-1
  Data Store Read19 : DataStoreRead  DataStoreName=ek11  SampleTime=-1
  Data Store Read2 : DataStoreRead  DataStoreName=Node2THETA  SampleTime=-1
  Data Store Read20 : DataStoreRead  DataStoreName=ksurf  SampleTime=-1
  Data Store Read21 : DataStoreRead  DataStoreName=ek11h  SampleTime=-1
  Data Store Read22 : DataStoreRead  DataStoreName=ek12  SampleTime=-1
  Data Store Read23 : DataStoreRead  DataStoreName=ek22  SampleTime=-1
  Data Store Read24 : DataStoreRead  DataStoreName=ek22h  SampleTime=-1
  Data Store Read25 : DataStoreRead  DataStoreName=fl  SampleTime=-1
  Data Store Read26 : DataStoreRead  DataStoreName=pmx  SampleTime=-1
  Data Store Read27 : DataStoreRead  DataStoreName=pr12  SampleTime=-1
  Data Store Read28 : DataStoreRead  DataStoreName=pr21  SampleTime=-1
  Data Store Read29 : DataStoreRead  DataStoreName=psh  SampleTime=-1
  Data Store Read30 : DataStoreRead  DataStoreName=sina  SampleTime=-1
  Data Store Read31 : DataStoreRead  DataStoreName=bmy  SampleTime=-1
  Data Store Read4 : DataStoreRead  DataStoreName=Node1UY  SampleTime=-1
  Data Store Read8 : DataStoreRead  DataStoreName=Node1THETA  SampleTime=-1
  Data Store Read9 : DataStoreRead  DataStoreName=Node2UX  SampleTime=-1
  Element : Outport  OutDataType=sfix(16)  OutScaling=2^0
  a1 : Outport  Port=2  OutDataType=sfix(16)  OutScaling=2^0
  a2 : Outport  Port=3  OutDataType=sfix(16)  OutScaling=2^0
  pmx : Outport  Port=4  OutDataType=sfix(16)  OutScaling=2^0
  bmy : Outport  Port=5  OutDataType=sfix(16)  OutScaling=2^0
  wires:
  Data Store Read2/1 -> Bus Creator/19
  Data Store Read13/1 -> Bus Creator/18
  Data Store Read9/1 -> Bus Creator/17
  Data Store Read8/1 -> Bus Creator/16
  Data Store Read4/1 -> Bus Creator/15
  Data Store Read1/1 -> Bus Creator/14
  Bus Creator/1 -> Element/1
  Data Store Read20/1 -> Bus Creator/1  "ksurf"
  Data Store Read17/1 -> Bus Creator/2  "cosa"
  Data Store Read18/1 -> Bus Creator/3  "eal"
  Data Store Read19/1 -> Bus Creator/4  "ek11"
  Data Store Read21/1 -> Bus Creator/5  "ek11h"
  Data Store Read22/1 -> Bus Creator/6  "ek12"
  Data Store Read23/1 -> Bus Creator/7  "ek22"
  Data Store Read24/1 -> Bus Creator/8  "ek22h"
  Data Store Read25/1 -> Bus Creator/9  "fl"
  Data Store Read27/1 -> Bus Creator/10  "pr12"
  Data Store Read28/1 -> Bus Creator/11  "pr21"
  Data Store Read29/1 -> Bus Creator/12  "psh"
  Data Store Read30/1 -> Bus Creator/13  "sina"
  Data Store Read15/1 -> a1/1  "a1"
  Data Store Read16/1 -> a2/1  "a2"
  Data Store Read26/1 -> pmx/1  "pmx"
  Data Store Read31/1 -> bmy/1  "bmy"

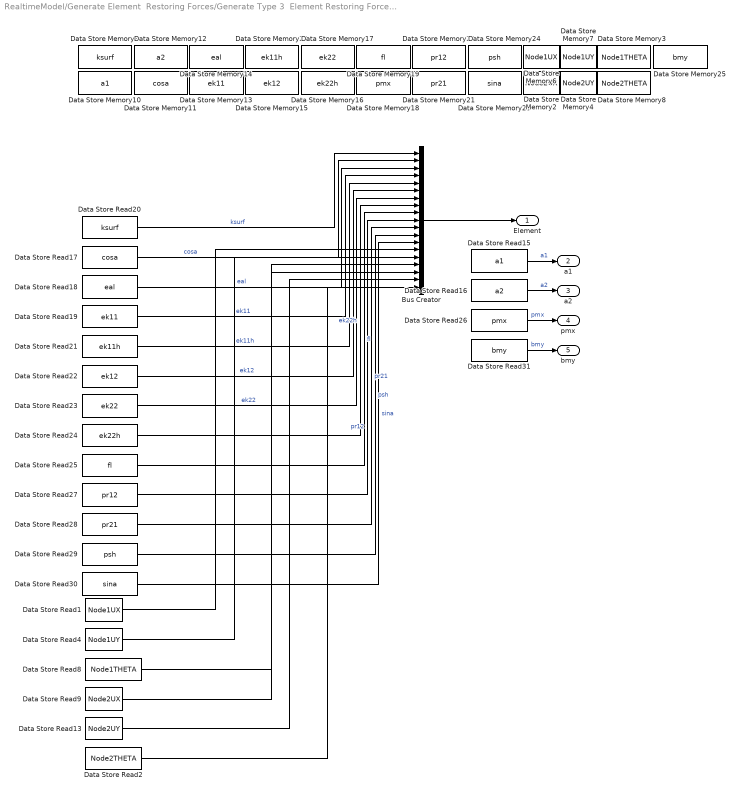
== system RealtimeModel/Generate Element  Restoring Forces/Generate Type 3  Element Restoring Force Element 2/Type 3 Element  ==
  Bus Creator : BusCreator  Inputs=19
  Data Store Memory10 : DataStoreMemory  DataStoreName=a1  InitialValue=Elements{id}.a1  OutDataType=sfix(16)  OutScaling=2^0
  Data Store Memory11 : DataStoreMemory  DataStoreName=cosa  InitialValue=Elements{id}.cosa  OutDataType=sfix(16)  OutScaling=2^0
  Data Store Memory12 : DataStoreMemory  DataStoreName=a2  InitialValue=Elements{id}.a2  OutDataType=sfix(16)  OutScaling=2^0
  Data Store Memory13 : DataStoreMemory  DataStoreName=ek11  InitialValue=Elements{id}.ek11  OutDataType=sfix(16)  OutScaling=2^0
  Data Store Memory14 : DataStoreMemory  DataStoreName=eal  InitialValue=Elements{id}.eal  OutDataType=sfix(16)  OutScaling=2^0
  Data Store Memory15 : DataStoreMemory  DataStoreName=ek12  InitialValue=Elements{id}.ek12  OutDataType=sfix(16)  OutScaling=2^0
  Data Store Memory16 : DataStoreMemory  DataStoreName=ek22h  InitialValue=Elements{id}.ek22h  OutDataType=sfix(16)  OutScaling=2^0
  Data Store Memory17 : DataStoreMemory  DataStoreName=ek22  InitialValue=Elements{id}.ek22  OutDataType=sfix(16)  OutScaling=2^0
  Data Store Memory18 : DataStoreMemory  DataStoreName=pmx  InitialValue=Elements{id}.pmx  OutDataType=sfix(16)  OutScaling=2^0
  Data Store Memory19 : DataStoreMemory  DataStoreName=fl  InitialValue=Elements{id}.fl  OutDataType=sfix(16)  OutScaling=2^0
  Data Store Memory2 : DataStoreMemory  DataStoreName=Node2UX  InitialValue=Elements{id}.Nodes(2).UX  OutDataType=sfix(16)  OutScaling=2^0
  Data Store Memory20 : DataStoreMemory  DataStoreName=ek11h  InitialValue=Elements{id}.ek11h  OutDataType=sfix(16)  OutScaling=2^0
  Data Store Memory21 : DataStoreMemory  DataStoreName=pr21  InitialValue=Elements{id}.pr21  OutDataType=sfix(16)  OutScaling=2^0
  Data Store Memory22 : DataStoreMemory  DataStoreName=pr12  InitialValue=Elements{id}.pr12  OutDataType=sfix(16)  OutScaling=2^0
  Data Store Memory23 : DataStoreMemory  DataStoreName=sina  InitialValue=Elements{id}.sina  OutDataType=sfix(16)  OutScaling=2^0
  Data Store Memory24 : DataStoreMemory  DataStoreName=psh  InitialValue=Elements{id}.psh  OutDataType=sfix(16)  OutScaling=2^0
  Data Store Memory25 : DataStoreMemory  DataStoreName=bmy  InitialValue=Elements{id}.bmy  OutDataType=sfix(16)  OutScaling=2^0
  Data Store Memory3 : DataStoreMemory  DataStoreName=Node1THETA  InitialValue=Elements{id}.Nodes(1).THETA  OutDataType=sfix(16)  OutScaling=2^0
  Data Store Memory4 : DataStoreMemory  DataStoreName=Node2UY  InitialValue=Elements{id}.Nodes(2).UY  OutDataType=sfix(16)  OutScaling=2^0
  Data Store Memory6 : DataStoreMemory  DataStoreName=Node1UX  InitialValue=Elements{id}.Nodes(1).UX  OutDataType=sfix(16)  OutScaling=2^0
  Data Store Memory7 : DataStoreMemory  DataStoreName=Node1UY  InitialValue=Elements{id}.Nodes(1).UY  OutDataType=sfix(16)  OutScaling=2^0
  Data Store Memory8 : DataStoreMemory  DataStoreName=Node2THETA  InitialValue=Elements{id}.Nodes(2).THETA  OutDataType=sfix(16)  OutScaling=2^0
  Data Store Memory9 : DataStoreMemory  DataStoreName=ksurf  InitialValue=Elements{id}.ksurf  OutDataType=sfix(16)  OutScaling=2^0
  Data Store Read1 : DataStoreRead  DataStoreName=Node1UX  SampleTime=-1
  Data Store Read13 : DataStoreRead  DataStoreName=Node2UY  SampleTime=-1
  Data Store Read15 : DataStoreRead  DataStoreName=a1  SampleTime=-1
  Data Store Read16 : DataStoreRead  DataStoreName=a2  SampleTime=-1
  Data Store Read17 : DataStoreRead  DataStoreName=cosa  SampleTime=-1
  Data Store Read18 : DataStoreRead  DataStoreName=eal  SampleTime=-1
  Data Store Read19 : DataStoreRead  DataStoreName=ek11  SampleTime=-1
  Data Store Read2 : DataStoreRead  DataStoreName=Node2THETA  SampleTime=-1
  Data Store Read20 : DataStoreRead  DataStoreName=ksurf  SampleTime=-1
  Data Store Read21 : DataStoreRead  DataStoreName=ek11h  SampleTime=-1
  Data Store Read22 : DataStoreRead  DataStoreName=ek12  SampleTime=-1
  Data Store Read23 : DataStoreRead  DataStoreName=ek22  SampleTime=-1
  Data Store Read24 : DataStoreRead  DataStoreName=ek22h  SampleTime=-1
  Data Store Read25 : DataStoreRead  DataStoreName=fl  SampleTime=-1
  Data Store Read26 : DataStoreRead  DataStoreName=pmx  SampleTime=-1
  Data Store Read27 : DataStoreRead  DataStoreName=pr12  SampleTime=-1
  Data Store Read28 : DataStoreRead  DataStoreName=pr21  SampleTime=-1
  Data Store Read29 : DataStoreRead  DataStoreName=psh  SampleTime=-1
  Data Store Read30 : DataStoreRead  DataStoreName=sina  SampleTime=-1
  Data Store Read31 : DataStoreRead  DataStoreName=bmy  SampleTime=-1
  Data Store Read4 : DataStoreRead  DataStoreName=Node1UY  SampleTime=-1
  Data Store Read8 : DataStoreRead  DataStoreName=Node1THETA  SampleTime=-1
  Data Store Read9 : DataStoreRead  DataStoreName=Node2UX  SampleTime=-1
  Element : Outport  OutDataType=sfix(16)  OutScaling=2^0
  a1 : Outport  Port=2  OutDataType=sfix(16)  OutScaling=2^0
  a2 : Outport  Port=3  OutDataType=sfix(16)  OutScaling=2^0
  pmx : Outport  Port=4  OutDataType=sfix(16)  OutScaling=2^0
  bmy : Outport  Port=5  OutDataType=sfix(16)  OutScaling=2^0
  wires:
  Data Store Read31/1 -> bmy/1  "bmy"
  Data Store Read26/1 -> pmx/1  "pmx"
  Data Store Read16/1 -> a2/1  "a2"
  Data Store Read15/1 -> a1/1  "a1"
  Data Store Read30/1 -> Bus Creator/13  "sina"
  Data Store Read29/1 -> Bus Creator/12  "psh"
  Data Store Read28/1 -> Bus Creator/11  "pr21"
  Data Store Read27/1 -> Bus Creator/10  "pr12"
  Data Store Read25/1 -> Bus Creator/9  "fl"
  Data Store Read24/1 -> Bus Creator/8  "ek22h"
  Data Store Read23/1 -> Bus Creator/7  "ek22"
  Data Store Read22/1 -> Bus Creator/6  "ek12"
  Data Store Read21/1 -> Bus Creator/5  "ek11h"
  Data Store Read19/1 -> Bus Creator/4  "ek11"
  Data Store Read18/1 -> Bus Creator/3  "eal"
  Data Store Read17/1 -> Bus Creator/2  "cosa"
  Data Store Read20/1 -> Bus Creator/1  "ksurf"
  Bus Creator/1 -> Element/1
  Data Store Read1/1 -> Bus Creator/14
  Data Store Read4/1 -> Bus Creator/15
  Data Store Read8/1 -> Bus Creator/16
  Data Store Read9/1 -> Bus Creator/17
  Data Store Read13/1 -> Bus Creator/18
  Data Store Read2/1 -> Bus Creator/19

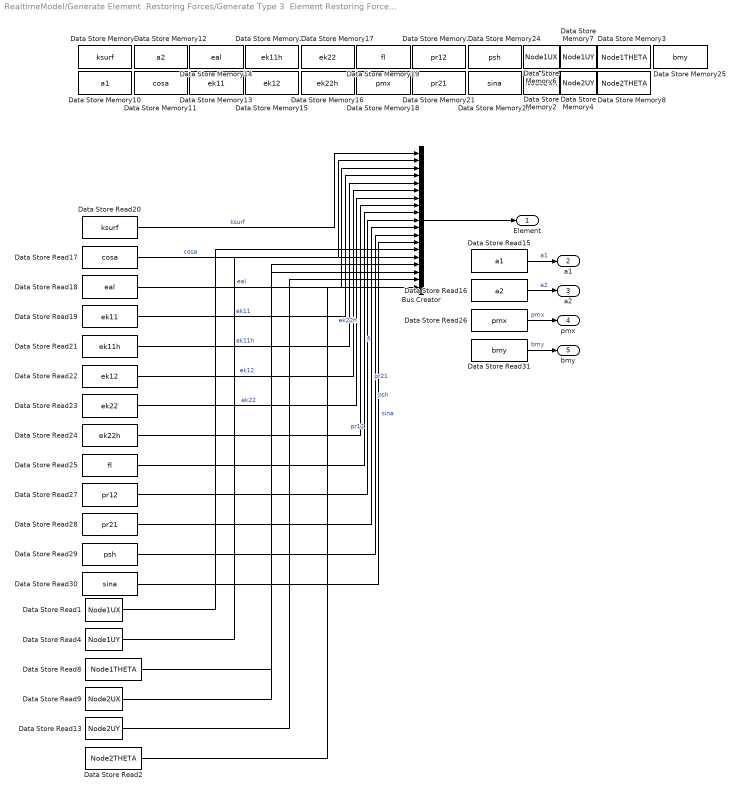
== system RealtimeModel/Generate Element  Restoring Forces/Generate Type 3  Element Restoring Force Element 4/Type 3 Element  ==
  Bus Creator : BusCreator  Inputs=19
  Data Store Memory10 : DataStoreMemory  DataStoreName=a1  InitialValue=Elements{id}.a1  OutDataType=sfix(16)  OutScaling=2^0
  Data Store Memory11 : DataStoreMemory  DataStoreName=cosa  InitialValue=Elements{id}.cosa  OutDataType=sfix(16)  OutScaling=2^0
  Data Store Memory12 : DataStoreMemory  DataStoreName=a2  InitialValue=Elements{id}.a2  OutDataType=sfix(16)  OutScaling=2^0
  Data Store Memory13 : DataStoreMemory  DataStoreName=ek11  InitialValue=Elements{id}.ek11  OutDataType=sfix(16)  OutScaling=2^0
  Data Store Memory14 : DataStoreMemory  DataStoreName=eal  InitialValue=Elements{id}.eal  OutDataType=sfix(16)  OutScaling=2^0
  Data Store Memory15 : DataStoreMemory  DataStoreName=ek12  InitialValue=Elements{id}.ek12  OutDataType=sfix(16)  OutScaling=2^0
  Data Store Memory16 : DataStoreMemory  DataStoreName=ek22h  InitialValue=Elements{id}.ek22h  OutDataType=sfix(16)  OutScaling=2^0
  Data Store Memory17 : DataStoreMemory  DataStoreName=ek22  InitialValue=Elements{id}.ek22  OutDataType=sfix(16)  OutScaling=2^0
  Data Store Memory18 : DataStoreMemory  DataStoreName=pmx  InitialValue=Elements{id}.pmx  OutDataType=sfix(16)  OutScaling=2^0
  Data Store Memory19 : DataStoreMemory  DataStoreName=fl  InitialValue=Elements{id}.fl  OutDataType=sfix(16)  OutScaling=2^0
  Data Store Memory2 : DataStoreMemory  DataStoreName=Node2UX  InitialValue=Elements{id}.Nodes(2).UX  OutDataType=sfix(16)  OutScaling=2^0
  Data Store Memory20 : DataStoreMemory  DataStoreName=ek11h  InitialValue=Elements{id}.ek11h  OutDataType=sfix(16)  OutScaling=2^0
  Data Store Memory21 : DataStoreMemory  DataStoreName=pr21  InitialValue=Elements{id}.pr21  OutDataType=sfix(16)  OutScaling=2^0
  Data Store Memory22 : DataStoreMemory  DataStoreName=pr12  InitialValue=Elements{id}.pr12  OutDataType=sfix(16)  OutScaling=2^0
  Data Store Memory23 : DataStoreMemory  DataStoreName=sina  InitialValue=Elements{id}.sina  OutDataType=sfix(16)  OutScaling=2^0
  Data Store Memory24 : DataStoreMemory  DataStoreName=psh  InitialValue=Elements{id}.psh  OutDataType=sfix(16)  OutScaling=2^0
  Data Store Memory25 : DataStoreMemory  DataStoreName=bmy  InitialValue=Elements{id}.bmy  OutDataType=sfix(16)  OutScaling=2^0
  Data Store Memory3 : DataStoreMemory  DataStoreName=Node1THETA  InitialValue=Elements{id}.Nodes(1).THETA  OutDataType=sfix(16)  OutScaling=2^0
  Data Store Memory4 : DataStoreMemory  DataStoreName=Node2UY  InitialValue=Elements{id}.Nodes(2).UY  OutDataType=sfix(16)  OutScaling=2^0
  Data Store Memory6 : DataStoreMemory  DataStoreName=Node1UX  InitialValue=Elements{id}.Nodes(1).UX  OutDataType=sfix(16)  OutScaling=2^0
  Data Store Memory7 : DataStoreMemory  DataStoreName=Node1UY  InitialValue=Elements{id}.Nodes(1).UY  OutDataType=sfix(16)  OutScaling=2^0
  Data Store Memory8 : DataStoreMemory  DataStoreName=Node2THETA  InitialValue=Elements{id}.Nodes(2).THETA  OutDataType=sfix(16)  OutScaling=2^0
  Data Store Memory9 : DataStoreMemory  DataStoreName=ksurf  InitialValue=Elements{id}.ksurf  OutDataType=sfix(16)  OutScaling=2^0
  Data Store Read1 : DataStoreRead  DataStoreName=Node1UX  SampleTime=-1
  Data Store Read13 : DataStoreRead  DataStoreName=Node2UY  SampleTime=-1
  Data Store Read15 : DataStoreRead  DataStoreName=a1  SampleTime=-1
  Data Store Read16 : DataStoreRead  DataStoreName=a2  SampleTime=-1
  Data Store Read17 : DataStoreRead  DataStoreName=cosa  SampleTime=-1
  Data Store Read18 : DataStoreRead  DataStoreName=eal  SampleTime=-1
  Data Store Read19 : DataStoreRead  DataStoreName=ek11  SampleTime=-1
  Data Store Read2 : DataStoreRead  DataStoreName=Node2THETA  SampleTime=-1
  Data Store Read20 : DataStoreRead  DataStoreName=ksurf  SampleTime=-1
  Data Store Read21 : DataStoreRead  DataStoreName=ek11h  SampleTime=-1
  Data Store Read22 : DataStoreRead  DataStoreName=ek12  SampleTime=-1
  Data Store Read23 : DataStoreRead  DataStoreName=ek22  SampleTime=-1
  Data Store Read24 : DataStoreRead  DataStoreName=ek22h  SampleTime=-1
  Data Store Read25 : DataStoreRead  DataStoreName=fl  SampleTime=-1
  Data Store Read26 : DataStoreRead  DataStoreName=pmx  SampleTime=-1
  Data Store Read27 : DataStoreRead  DataStoreName=pr12  SampleTime=-1
  Data Store Read28 : DataStoreRead  DataStoreName=pr21  SampleTime=-1
  Data Store Read29 : DataStoreRead  DataStoreName=psh  SampleTime=-1
  Data Store Read30 : DataStoreRead  DataStoreName=sina  SampleTime=-1
  Data Store Read31 : DataStoreRead  DataStoreName=bmy  SampleTime=-1
  Data Store Read4 : DataStoreRead  DataStoreName=Node1UY  SampleTime=-1
  Data Store Read8 : DataStoreRead  DataStoreName=Node1THETA  SampleTime=-1
  Data Store Read9 : DataStoreRead  DataStoreName=Node2UX  SampleTime=-1
  Element : Outport  OutDataType=sfix(16)  OutScaling=2^0
  a1 : Outport  Port=2  OutDataType=sfix(16)  OutScaling=2^0
  a2 : Outport  Port=3  OutDataType=sfix(16)  OutScaling=2^0
  pmx : Outport  Port=4  OutDataType=sfix(16)  OutScaling=2^0
  bmy : Outport  Port=5  OutDataType=sfix(16)  OutScaling=2^0
  wires:
  Data Store Read2/1 -> Bus Creator/19
  Data Store Read13/1 -> Bus Creator/18
  Data Store Read9/1 -> Bus Creator/17
  Data Store Read8/1 -> Bus Creator/16
  Data Store Read4/1 -> Bus Creator/15
  Data Store Read1/1 -> Bus Creator/14
  Bus Creator/1 -> Element/1
  Data Store Read20/1 -> Bus Creator/1  "ksurf"
  Data Store Read17/1 -> Bus Creator/2  "cosa"
  Data Store Read18/1 -> Bus Creator/3  "eal"
  Data Store Read19/1 -> Bus Creator/4  "ek11"
  Data Store Read21/1 -> Bus Creator/5  "ek11h"
  Data Store Read22/1 -> Bus Creator/6  "ek12"
  Data Store Read23/1 -> Bus Creator/7  "ek22"
  Data Store Read24/1 -> Bus Creator/8  "ek22h"
  Data Store Read25/1 -> Bus Creator/9  "fl"
  Data Store Read27/1 -> Bus Creator/10  "pr12"
  Data Store Read28/1 -> Bus Creator/11  "pr21"
  Data Store Read29/1 -> Bus Creator/12  "psh"
  Data Store Read30/1 -> Bus Creator/13  "sina"
  Data Store Read15/1 -> a1/1  "a1"
  Data Store Read16/1 -> a2/1  "a2"
  Data Store Read26/1 -> pmx/1  "pmx"
  Data Store Read31/1 -> bmy/1  "bmy"
